simulink model "AMPC_CSimNN_SysIdent"  (R2019a)
settings: Solver=VariableStepAuto  StartTime=0.0  StopTime=15  FixedStep=0.025  RelTol=1e-4
libraries: neural x62, mpclib x2
(part 3 of 3)

== matlab function AMPC_CSimNN_SysIdent/MATLAB Function2 ==
  data: Vx input; A output size=[2,2]; Cf input; Cr input; steer input; x input size=[2,1]; B output size=[2,1]; C output size=[2,2]; D output size=[2,1]; U output size=1; Y output size=[2,1]; X output size=[2,1]; DX output size=[2,1]
function [A,B,C,D,U,Y,X,DX] = fcn(Vx,Cf,Cr,steer,x)
% Sample time
Ts = 0.025;

% Model parameters
m = 1650;
Iz = 3234;
lf = 1.4;
lr = 1.65;

% Continuous-time model
Ac=[-(Cf+Cr)/(m*Vx), -1-(lf*Cf-lr*Cr)/(m*Vx^2);
    -(lf*Cf-lr*Cr)/Iz, -(lf^2*Cf+lr^2*Cr)/(Iz*Vx)];

Bc=[Cf/(m*Vx);(lf*Cf)/Iz];

Cc=eye(2);

Dc=zeros(2,1);

% Generate discrete-time model
nx = size(Ac,1);
nu = size(Bc,2);
M = expm([[Ac Bc]*Ts; zeros(nu,nx+nu)]);
A = M(1:nx,1:nx);
B = M(1:nx,nx+1:nx+nu);
C = Cc;
D = Dc;

% Nominal conditions for discrete-time plant
X = x;
U = steer;
Y = C*x + D*steer;
DX = A*x+B*steer-x;

== matlab function AMPC_CSimNN_SysIdent/MATLAB Function1 ==
  data: Vx input; A output size=[2,2]; Cf input; Cr input; steer input; x input size=[2,1]; B output size=[2,1]; C output size=[2,2]; D output size=[2,1]; U output size=1; Y output size=[2,1]; X output size=[2,1]; DX output size=[2,1]
function [A,B,C,D,U,Y,X,DX] = fcn(Vx,Cf,Cr,steer,x)
% Sample time
Ts = 0.025;

% Model parameters
m = 1650;
Iz = 3234;
lf = 1.4;
lr = 1.65;

% Continuous-time model
Ac=[-(Cf+Cr)/(m*Vx), -1-(lf*Cf-lr*Cr)/(m*Vx^2);
    -(lf*Cf-lr*Cr)/Iz, -(lf^2*Cf+lr^2*Cr)/(Iz*Vx)];

Bc=[Cf/(m*Vx);(lf*Cf)/Iz];

Cc=eye(2);

Dc=zeros(2,1);

% Generate discrete-time model
nx = size(Ac,1);
nu = size(Bc,2);
M = expm([[Ac Bc]*Ts; zeros(nu,nx+nu)]);
A = M(1:nx,1:nx);
B = M(1:nx,nx+1:nx+nu);
C = Cc;
D = Dc;

% Nominal conditions for discrete-time plant
X = x;
U = steer;
Y = C*x + D*steer;
DX = A*x+B*steer-x;
